simulink model "modelo_int_deriv"  (R2016a)
settings: Solver=FixedStepAuto  StartTime=0.0  StopTime=100  FixedStep=0.0001  RelTol=1e-3
settings Model: Creator=itsaso  LastModifiedBy=itsaso

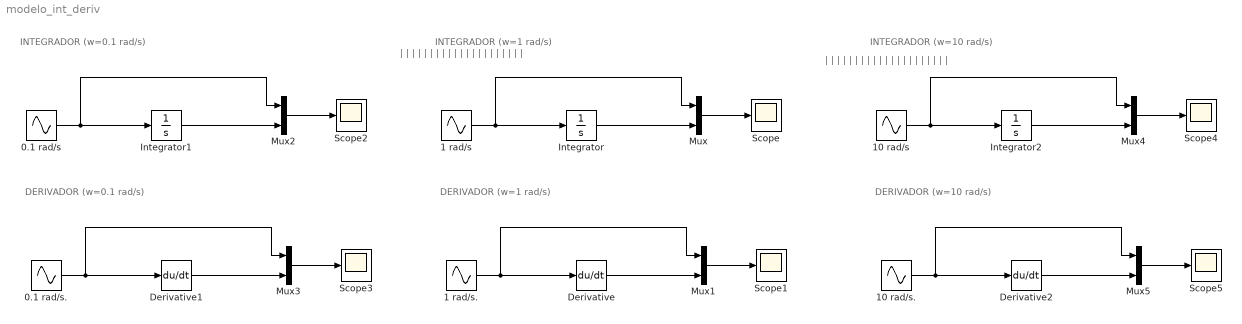
== system modelo_int_deriv ==
  note: |
      | |
      | |
      | |
      | |
      | |
      | |
      | |
      | |
      | |
      | |
      | |
      | |
      | |
      | |
      | |
      | |
      | |
      | |
      | |
      | |
  note: INTEGRADOR (w=1 rad/s)
  note: DERIVADOR (w=1 rad/s)
  note: INTEGRADOR (w=0.1 rad/s)
  note: DERIVADOR (w=0.1 rad/s)
  note: INTEGRADOR (w=10 rad/s)
  note: DERIVADOR (w=10 rad/s)
  note: |
      | |
      | |
      | |
      | |
      | |
      | |
      | |
      | |
      | |
      | |
      | |
      | |
      | |
      | |
      | |
      | |
      | |
      | |
      | |
      | |
  0.1 rad/s : Sin  Frequency=0.1  Phase=pi/2  SampleTime=0
  0.1 rad/s. : Sin  Frequency=0.1  Phase=pi/2  SampleTime=0
  1 rad/s : Sin  Frequency=1*1  Phase=pi/2  SampleTime=0
  1 rad/s. : Sin  Frequency=1*1  Phase=pi/2  SampleTime=0
  10 rad/s : Sin  Frequency=10  Phase=pi/2  SampleTime=0
  10 rad/s. : Sin  Frequency=10  Phase=pi/2  SampleTime=0
  Derivative : Derivative
  Derivative1 : Derivative
  Derivative2 : Derivative
  Integrator : Integrator
  Integrator1 : Integrator
  Integrator2 : Integrator
  Mux{,1..5} (6 alike) : Mux  Inputs=2
  Scope{,1..5} (6 alike) : Scope
  wires:
  1 rad/s/1 -> Mux/1, Integrator/1
  Integrator/1 -> Mux/2
  Mux/1 -> Scope/1
  1 rad/s./1 -> Derivative/1, Mux1/1
  Derivative/1 -> Mux1/2
  Mux1/1 -> Scope1/1
  0.1 rad/s/1 -> Integrator1/1, Mux2/1
  Integrator1/1 -> Mux2/2
  Mux2/1 -> Scope2/1
  0.1 rad/s./1 -> Mux3/1, Derivative1/1
  Derivative1/1 -> Mux3/2
  Mux3/1 -> Scope3/1
  10 rad/s/1 -> Integrator2/1, Mux4/1
  Integrator2/1 -> Mux4/2
  Mux4/1 -> Scope4/1
  10 rad/s./1 -> Mux5/1, Derivative2/1
  Derivative2/1 -> Mux5/2
  Mux5/1 -> Scope5/1
